simulink model "FrankSensingDiscreteEKF"  (R2025a)
settings: Solver=FixedStepAuto  StartTime=0.0  StopTime=150  FixedStep=.001  RelTol=1e-3
model workspace (MAT data in the model file):
  GPSvehyUpdate = 0
libraries: simulink x1
(part 1 of 2)
settings Model: SimulationMode=rapid-accelerator  Creator=ncpet  LastModifiedBy=ncpet
settings RTWCC: GPUComputeCapability=3.5

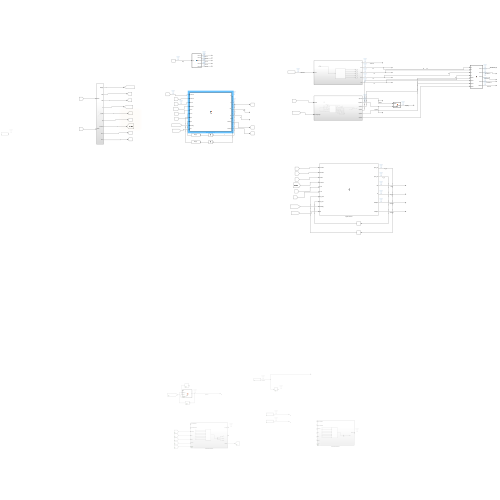
[thumbnail: Simulink's stored preview of the top-level diagram]
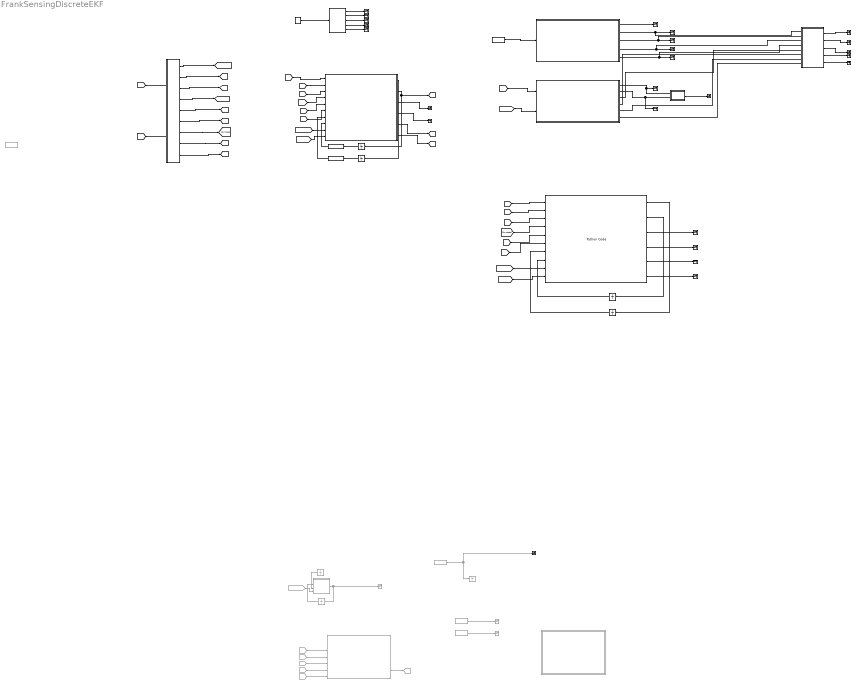
== system FrankSensingDiscreteEKF ==
  From Workspace : FromWorkspace  VariableName=LatAccel
  From Workspace4 : FromWorkspace  Commented=on  VariableName=X
  From Workspace5 : FromWorkspace  Commented=on  VariableName=Y
  From Workspace6 : FromWorkspace  Commented=on  VariableName=SteeringAngle
  From Workspace8 : FromWorkspace  Commented=on  VariableName=TicksYR
  From14 : From  Commented=on  GotoTag=startflag
  From3 : From  Commented=on  GotoTag=Vvehx
  From4 : From  Commented=on  GotoTag=Steerangle
  From5 : From  Commented=on  GotoTag=Psid
  From6 : From  Commented=on  GotoTag=Xcov
  From7 : From  Commented=on  GotoTag=Ycov
  Goto5 : Goto  Commented=on  GotoTag=Rbias
  Integrator1 : Integrator  Commented=on
  MATLAB Function : MATLAB Function  Commented=on  TreatAsAtomicUnit=on
  MATLAB Function1 : MATLAB Function  TreatAsAtomicUnit=on
  MATLAB Function2 : MATLAB Function  TreatAsAtomicUnit=on
  MATLAB Function3 : MATLAB Function  TreatAsAtomicUnit=on
  MATLAB Function4 : MATLAB Function  TreatAsAtomicUnit=on
  Python Code1 : PythonCode  InitializeConditionsCode=|  OutputCode=|  TerminateCode=pass  SampleTime=.001
      InitializeConditionsCode=|
      | import numpy as np
      | 
      | # Initial state vector  [Vy, Vx, r, Psi, Ax, Rbias, Abias]
      | Xpri_init = np.array([0.5, -1.9, -0.49, 0.0, 0.34, -0.022, -0.2], dtype=float)
      | 
      | # Initial covariance (7x7 diagonal), flattened row-major
      | P_init_diag = np.diag([0.1, 0.1, 0.1, 0.1, 0.001, 0.001, 0.001])
      | Ppri_init   = P_init_diag.flatten()   # 49 values
      OutputCode=|
      | import numpy as np
      | import EKFfcn2
      | 
      | u = [VYmeas, VXmeas, rmeas, Axmeas,
      |      Xcov, Ycov,
      |      *Ppri_flat,   # 49 values (7x7 flattened)
      |      *Xpri_arr,    # 7 values
      |      startflag,
      |      SA]
      | 
      | y = EKFfcn2.simulink_step(u)
      | 
      | # Unpack outputs
      | Ppri_out  = y[0:49]    # 7x7 covariance, flattened
      | Xpri_out  = y[49:56]   # 7 states
      | res       = y[56:60]   # 4 residuals
      | fk        = y[60:67]   # 7 predicted states
      | Rbiaspri  = y[67]
      | Abiaspri  = y[68]
  Ramp : simulink/Sources/Ramp  slope=.1  start=0  InitialOutput=.001
  Signal Specification : SignalSpecification  Dimensions=[7 7]
  Signal Specification1 : SignalSpecification  Dimensions=[7 1]
  State Estimation : Subsystem  Commented=on
  State Estimation1 : Subsystem  Commented=on
  Subsystem1 : Subsystem
  Subsystem3 : Subsystem
  Subsystem4 : Subsystem
  Terminator : Terminator  Commented=on
  Terminator{1..2,5..23,29..32} (25 alike) : Terminator
  Terminator3 : Terminator  Commented=on
  Terminator4 : Terminator  Commented=on
  Unit Delay : UnitDelay  Commented=on  SampleTime=-1  HasFrameUpgradeWarning=on
  Unit Delay1 : UnitDelay  Commented=on  SampleTime=-1  HasFrameUpgradeWarning=on
  Unit Delay2 : UnitDelay  SampleTime=-1  HasFrameUpgradeWarning=on
  Unit Delay3 : UnitDelay  InitialCondition=[.1 0 0 0 0 0 0, 0 .1 0 0 0 0 0, 0 0 .1 0 0 0 0, 0 0 0 .1 0 0 0, 0 0 0 0 .001 0 0, 0 0 0 0 0 .001 0, 0 0 0 0 0 0 .001]  SampleTime=.001  HasFrameUpgradeWarning=on
  Unit Delay4 : UnitDelay  SampleTime=-1  HasFrameUpgradeWarning=on
  Unit Delay5 : UnitDelay  InitialCondition=[.5, -1.9, -.49, 0, .34, -.022, -.2]  SampleTime=.001  HasFrameUpgradeWarning=on
  wires:
  From Workspace4/1 -> Terminator3/1  "x"
  From Workspace5/1 -> Terminator4/1  "y"
  From Workspace8/1 -> Integrator1/1, Terminator13/1  "TicksYR"
  From3/1 -> State Estimation/4(Vx)
  From4/1 -> State Estimation/5(SA)
  From5/1 -> State Estimation/3(rmeas)
  From6/1 -> State Estimation/6(Xcov)
  From7/1 -> State Estimation/7(Ycov)
  State Estimation/3(Rbias) -> Goto5/1
  MATLAB Function/1(x) -> Terminator/1, Unit Delay/1  "psiNum"
  Unit Delay/1 -> MATLAB Function/2(Xdpri)
  From14/1 -> MATLAB Function/4(startflag)
  Unit Delay1/1 -> MATLAB Function/3(Xpri)
  Subsystem1/1(Slipflag) -> [startflag]
  Subsystem1/2(XdS) -> [Xd]
  Subsystem1/3(YdS) -> [Yd]
  Subsystem1/4(Out4) -> [Steerangle]
  Subsystem1/5(PsidS) -> [Psid]
  Subsystem1/6(psi) -> [psi]
  Subsystem1/7(Axmeas) -> [Axmeas]
  Subsystem1/8(Xcov) -> [Xcov]
  Subsystem1/9(Ycov) -> [Ycov]
  [Xcov] -> MATLAB Function1/5(Xcov)
  [Ycov] -> MATLAB Function1/6(Ycov)
  MATLAB Function1/2(X) -> Unit Delay2/1, [States]  "X"
  Unit Delay2/1 -> Signal Specification1/1
  MATLAB Function1/1(P) -> Unit Delay4/1  "Pmat"
  Unit Delay4/1 -> Signal Specification/1
  [Axmeas] -> MATLAB Function1/4(Axmeas)
  [Xd] -> MATLAB Function1/2(VXmeas)
  [startflag] -> MATLAB Function1/9(startflag)
  [Steerangle] -> MATLAB Function1/10(SA)
  Signal Specification/1 -> MATLAB Function1/7(Ppri)
  Signal Specification1/1 -> MATLAB Function1/8(Xpri)
  MATLAB Function1/3(res) -> Terminator1/1  "res"
  MATLAB Function1/4(fk) -> Terminator2/1  "fk"
  [States] -> Subsystem3/1(States)
  [Steerangle] -> Subsystem3/2(SteeringAngle)
  Subsystem3/1(AlphaF) -> MATLAB Function2/1(AlphaF), Terminator5/1  "AlphaF"
  Subsystem3/2(AlphaR) -> Terminator8/1, MATLAB Function2/2(AlphaR)  "AlphaR"
  MATLAB Function2/1(SlipMag) -> Terminator10/1  "SlipMag"
  From Workspace/1 -> Subsystem4/1(Accel)  "LatAccel"
  Subsystem4/1(Outport) -> Terminator11/1  "TireForce"
  MATLAB Function1/5(Rbiaspri) -> [Rbias]
  [Rbias] -> Subsystem1/1(Rbias)
  MATLAB Function1/6(Abiaspri) -> [Abiaspri]
  [Abiaspri] -> Subsystem1/2(Abias)
  Ramp/1 -> MATLAB Function3/1(slip)  "Slip"
  MATLAB Function3/1(Force1) -> Terminator14/1  "Force1"
  MATLAB Function3/2(Force2) -> Terminator15/1  "Force2"
  MATLAB Function3/3(Force3) -> Terminator16/1  "Force3"
  MATLAB Function3/5(Force5) -> Terminator18/1  "Force5"
  MATLAB Function3/4(Force4) -> Terminator17/1  "Force4"
  Subsystem3/5(Alpha4) -> MATLAB Function4/7(Alpha4)
  Subsystem4/3(Ffl) -> MATLAB Function4/2(Ffl), Terminator7/1  "Ffl"
  MATLAB Function4/5(TotForce) -> Terminator23/1  "TotForce"
  MATLAB Function4/2(Force2) -> Terminator20/1  "FflLatForce"
  Subsystem3/4(Alpha3) -> MATLAB Function4/6(Alpha3)
  Subsystem4/4(Frr) -> MATLAB Function4/3(Frr), Terminator9/1  "Frr"
  Subsystem3/6(Alpha5) -> MATLAB Function4/8(Alpha5)
  Subsystem3/3(Alpha2) -> MATLAB Function4/5(Alpha2)
  MATLAB Function4/4(Force4) -> Terminator22/1  "FrlLatForce"
  MATLAB Function4/1(Force1) -> Terminator19/1  "FfrLatForce"
  Subsystem4/5(Frl) -> MATLAB Function4/4(Frl), Terminator12/1  "Frl"
  Subsystem4/2(Ffr) -> MATLAB Function4/1(Ffr), Terminator6/1  "Ffr"
  MATLAB Function4/3(Force3) -> Terminator21/1  "FrrLatForce"
  Unit Delay3/1 -> Python Code1/7
  Python Code1/1 -> Unit Delay3/1  "P_py"
  Python Code1/2 -> Unit Delay5/1  "X_py"
  Unit Delay5/1 -> Python Code1/8
  [startflag] -> Python Code1/9
  Python Code1/6 -> Terminator32/1  "AbiasPY"
  Python Code1/5 -> Terminator31/1  "RbiasPY"
  Python Code1/4 -> Terminator30/1  "fk_py"
  Python Code1/3 -> Terminator29/1  "resPY"
  [Axmeas] -> Python Code1/4
  [Psid] -> Python Code1/3
  [Xd] -> Python Code1/2
  [Ycov] -> Python Code1/6
  [Xcov] -> Python Code1/5
  [Yd] -> Python Code1/1
  [Steerangle] -> Python Code1/10
  [Yd] -> MATLAB Function1/1(VYmeas)
  [Psid] -> MATLAB Function1/3(rmeas)

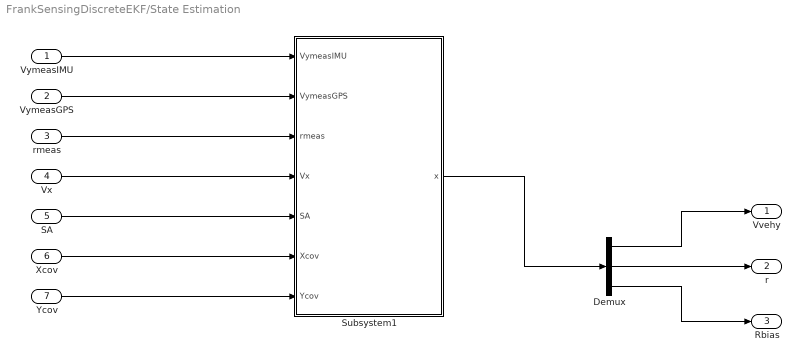
== system FrankSensingDiscreteEKF/State Estimation ==
  VymeasIMU : Inport
  VymeasGPS : Inport  Port=2
  rmeas : Inport  Port=3
  Vx : Inport  Port=4
  SA : Inport  Port=5
  Xcov : Inport  Port=6
  Ycov : Inport  Port=7
  Demux : Demux  Outputs=3
  Subsystem1 : Subsystem
  Vvehy : Outport
  r : Outport  Port=2
  Rbias : Outport  Port=3
  wires:
  VymeasIMU/1 -> Subsystem1/1(VymeasIMU)
  VymeasGPS/1 -> Subsystem1/2(VymeasGPS)
  rmeas/1 -> Subsystem1/3(rmeas)
  Vx/1 -> Subsystem1/4(Vx)
  SA/1 -> Subsystem1/5(SA)
  Subsystem1/1(x) -> Demux/1
  Demux/1 -> Vvehy/1
  Xcov/1 -> Subsystem1/6(Xcov)
  Ycov/1 -> Subsystem1/7(Ycov)
  Demux/2 -> r/1
  Demux/3 -> Rbias/1

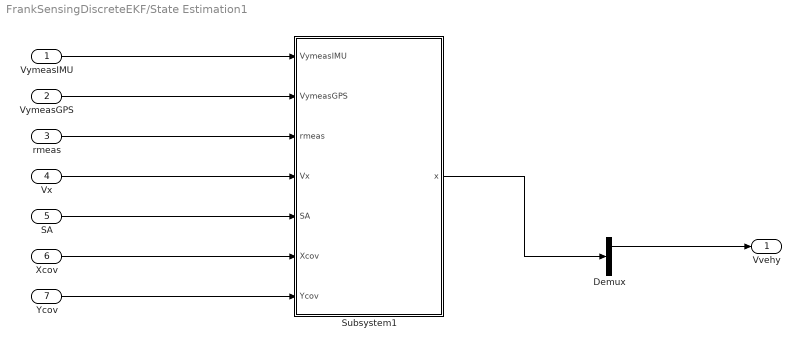
== system FrankSensingDiscreteEKF/State Estimation1 ==
  VymeasIMU : Inport
  VymeasGPS : Inport  Port=2
  rmeas : Inport  Port=3
  Vx : Inport  Port=4
  SA : Inport  Port=5
  Xcov : Inport  Port=6
  Ycov : Inport  Port=7
  Demux : Demux  Outputs=2
  Subsystem1 : Subsystem
  Vvehy : Outport
  wires:
  Ycov/1 -> Subsystem1/7(Ycov)
  Xcov/1 -> Subsystem1/6(Xcov)
  Demux/1 -> Vvehy/1
  Subsystem1/1(x) -> Demux/1
  SA/1 -> Subsystem1/5(SA)
  Vx/1 -> Subsystem1/4(Vx)
  rmeas/1 -> Subsystem1/3(rmeas)
  VymeasGPS/1 -> Subsystem1/2(VymeasGPS)
  VymeasIMU/1 -> Subsystem1/1(VymeasIMU)

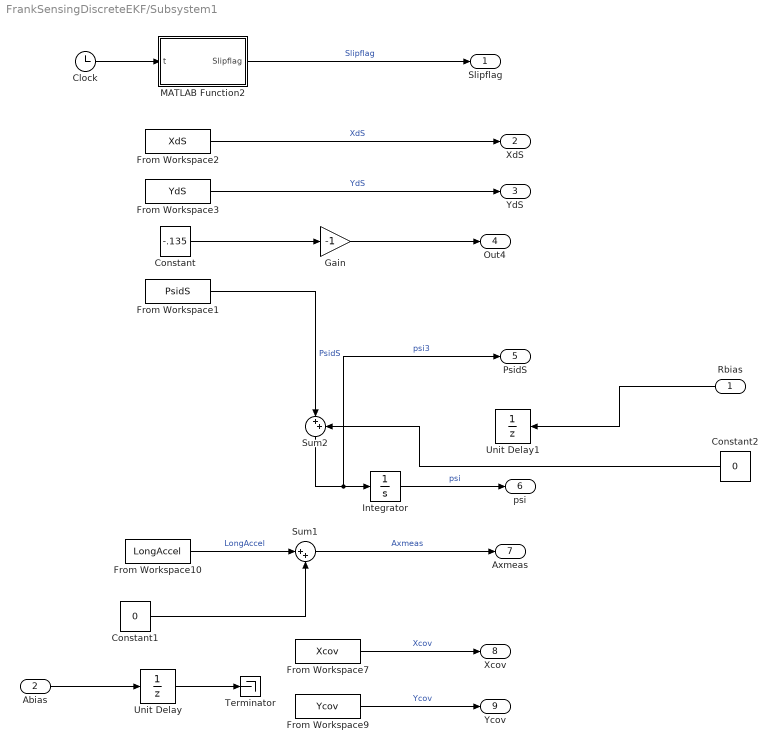
== system FrankSensingDiscreteEKF/Subsystem1 ==
  Rbias : Inport
  Abias : Inport  Port=2
  Clock : Clock
  Constant : Constant  Value=-.135
  Constant1 : Constant  Value=0
  Constant2 : Constant  Value=0
  From Workspace1 : FromWorkspace  VariableName=PsidS
  From Workspace10 : FromWorkspace  VariableName=LongAccel
  From Workspace2 : FromWorkspace  VariableName=XdS
  From Workspace3 : FromWorkspace  VariableName=YdS
  From Workspace7 : FromWorkspace  VariableName=Xcov
  From Workspace9 : FromWorkspace  VariableName=Ycov
  Gain : Gain  Gain=-1
  Integrator : Integrator
  MATLAB Function2 : MATLAB Function  TreatAsAtomicUnit=on
  Sum1 : Sum  Inputs=|++
  Sum2 : Sum  Inputs=|++
  Terminator : Terminator
  Unit Delay : UnitDelay  SampleTime=-1  HasFrameUpgradeWarning=on
  Unit Delay1 : UnitDelay  SampleTime=-1  HasFrameUpgradeWarning=on
  Slipflag : Outport
  XdS : Outport  Port=2
  YdS : Outport  Port=3
  Out4 : Outport  Port=4
  PsidS : Outport  Port=5
  psi : Outport  Port=6
  Axmeas : Outport  Port=7
  Xcov : Outport  Port=8
  Ycov : Outport  Port=9
  wires:
  From Workspace1/1 -> Sum2/1  "PsidS"
  From Workspace7/1 -> Xcov/1  "Xcov"
  Constant/1 -> Gain/1
  Sum2/1 -> PsidS/1, Integrator/1  "psi3"
  From Workspace10/1 -> Sum1/1  "LongAccel"
  Clock/1 -> MATLAB Function2/1(t)
  From Workspace9/1 -> Ycov/1  "Ycov"
  From Workspace2/1 -> XdS/1  "XdS"
  From Workspace3/1 -> YdS/1  "YdS"
  Integrator/1 -> psi/1  "psi"
  Sum1/1 -> Axmeas/1  "Axmeas"
  MATLAB Function2/1(Slipflag) -> Slipflag/1  "Slipflag"
  Abias/1 -> Unit Delay/1
  Rbias/1 -> Unit Delay1/1
  Gain/1 -> Out4/1
  Constant1/1 -> Sum1/2
  Unit Delay/1 -> Terminator/1
  Constant2/1 -> Sum2/2

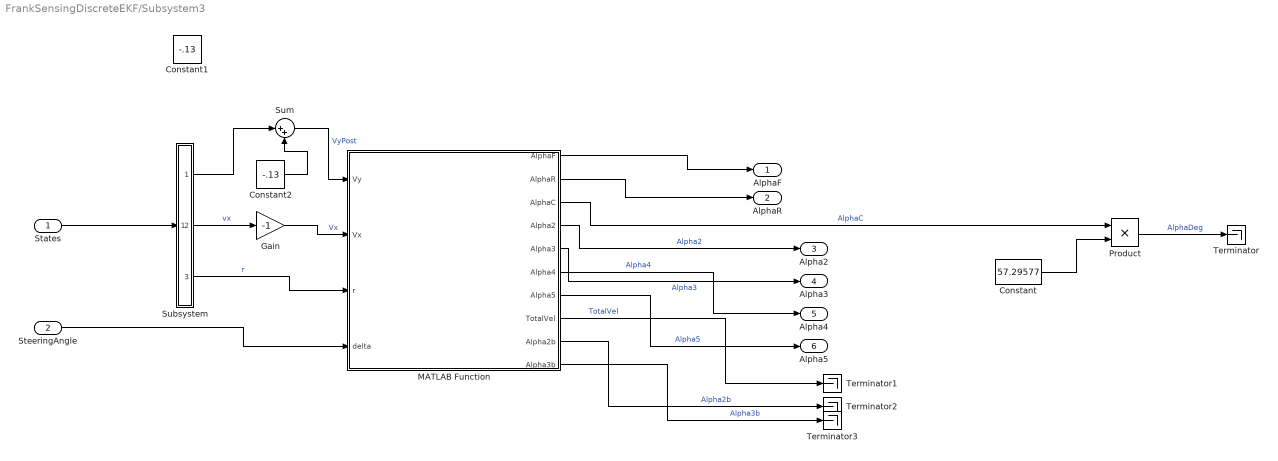
== system FrankSensingDiscreteEKF/Subsystem3 ==
  States : Inport
  SteeringAngle : Inport  Port=2
  Constant : Constant  Value=57.29577
  Constant1 : Constant  Value=-.13
  Constant2 : Constant  Value=-.13
  Gain : Gain  Gain=-1
  MATLAB Function : MATLAB Function  TreatAsAtomicUnit=on
  Product : Product
  Subsystem : Subsystem
  Sum : Sum  Inputs=|++
  Terminator{,1..3} (4 alike) : Terminator
  AlphaF : Outport
  AlphaR : Outport  Port=2
  Alpha2 : Outport  Port=3
  Alpha3 : Outport  Port=4
  Alpha4 : Outport  Port=5
  Alpha5 : Outport  Port=6
  wires:
  States/1 -> Subsystem/1(In1)
  Subsystem/2(Out2) -> Gain/1  "vx"
  Subsystem/3(Out3) -> MATLAB Function/3(r)  "r"
  SteeringAngle/1 -> MATLAB Function/4(delta)
  MATLAB Function/2(AlphaR) -> AlphaR/1
  MATLAB Function/1(AlphaF) -> AlphaF/1
  MATLAB Function/3(AlphaC) -> Product/1  "AlphaC"
  Constant/1 -> Product/2
  Product/1 -> Terminator/1  "AlphaDeg"
  MATLAB Function/4(Alpha2) -> Alpha2/1  "Alpha2"
  MATLAB Function/5(Alpha3) -> Alpha3/1  "Alpha3"
  MATLAB Function/6(Alpha4) -> Alpha4/1  "Alpha4"
  MATLAB Function/7(Alpha5) -> Alpha5/1  "Alpha5"
  MATLAB Function/8(TotalVel) -> Terminator1/1  "TotalVel"
  MATLAB Function/9(Alpha2b) -> Terminator2/1  "Alpha2b"
  MATLAB Function/10(Alpha3b) -> Terminator3/1  "Alpha3b"
  Gain/1 -> MATLAB Function/2(Vx)  "Vx"
  Subsystem/1(Out1) -> Sum/1
  Sum/1 -> MATLAB Function/1(Vy)  "VyPost"
  Constant2/1 -> Sum/2

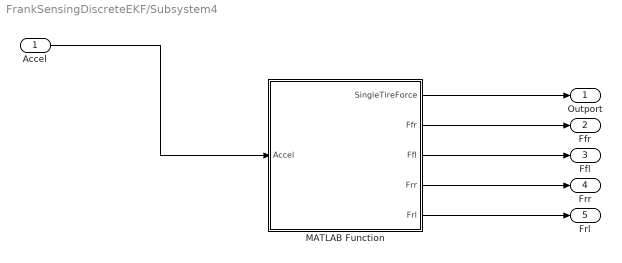
== system FrankSensingDiscreteEKF/Subsystem4 ==
  Accel : Inport
  MATLAB Function : MATLAB Function  TreatAsAtomicUnit=on
  Outport : Outport
  Ffr : Outport  Port=2
  Ffl : Outport  Port=3
  Frr : Outport  Port=4
  Frl : Outport  Port=5
  wires:
  Accel/1 -> MATLAB Function/1(Accel)
  MATLAB Function/1(SingleTireForce) -> Outport/1
  MATLAB Function/2(Ffr) -> Ffr/1
  MATLAB Function/3(Ffl) -> Ffl/1
  MATLAB Function/4(Frr) -> Frr/1
  MATLAB Function/5(Frl) -> Frl/1

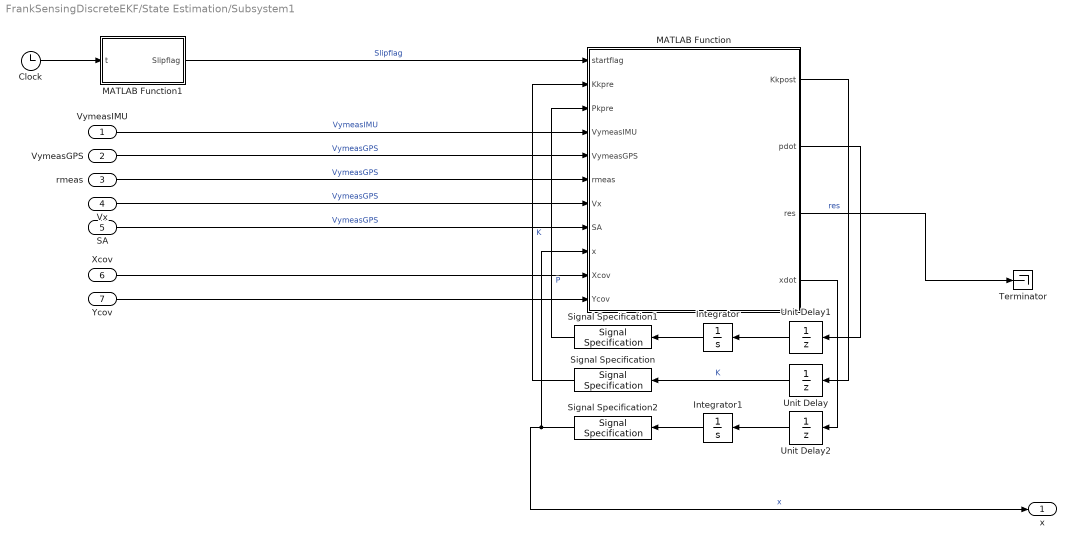
== system FrankSensingDiscreteEKF/State Estimation/Subsystem1 ==
  VymeasIMU : Inport
  VymeasGPS : Inport  Port=2
  rmeas : Inport  Port=3
  Vx : Inport  Port=4
  SA : Inport  Port=5
  Xcov : Inport  Port=6
  Ycov : Inport  Port=7
  Clock : Clock
  Integrator : Integrator  InitialCondition=[.001 0 0;0 .001 0;0 0 .001]
  Integrator1 : Integrator  InitialCondition=[-0.014;-0.44;-.022]
  MATLAB Function : MATLAB Function  TreatAsAtomicUnit=on
  MATLAB Function1 : MATLAB Function  TreatAsAtomicUnit=on
  Signal Specification : SignalSpecification  Dimensions=[3 3]
  Signal Specification1 : SignalSpecification  Dimensions=[3 3]
  Signal Specification2 : SignalSpecification  Dimensions=[3 1]
  Terminator : Terminator
  Unit Delay : UnitDelay  SampleTime=-1  HasFrameUpgradeWarning=on
  Unit Delay1 : UnitDelay  SampleTime=-1  HasFrameUpgradeWarning=on
  Unit Delay2 : UnitDelay  SampleTime=-1  HasFrameUpgradeWarning=on
  x : Outport
  wires:
  MATLAB Function/1(Kkpost) -> Unit Delay/1
  Signal Specification/1 -> MATLAB Function/2(Kkpre)  "K"
  MATLAB Function/2(pdot) -> Unit Delay1/1
  Integrator/1 -> Signal Specification1/1
  Unit Delay/1 -> Signal Specification/1  "K"
  Unit Delay1/1 -> Integrator/1
  Signal Specification1/1 -> MATLAB Function/3(Pkpre)  "P"
  VymeasIMU/1 -> MATLAB Function/4(VymeasIMU)  "VymeasIMU"
  MATLAB Function/3(res) -> Terminator/1  "res"
  VymeasGPS/1 -> MATLAB Function/5(VymeasGPS)  "VymeasGPS"
  rmeas/1 -> MATLAB Function/6(rmeas)  "VymeasGPS"
  Vx/1 -> MATLAB Function/7(Vx)  "VymeasGPS"
  Clock/1 -> MATLAB Function1/1(t)
  MATLAB Function1/1(Slipflag) -> MATLAB Function/1(startflag)  "Slipflag"
  SA/1 -> MATLAB Function/8(SA)  "VymeasGPS"
  MATLAB Function/4(xdot) -> Unit Delay2/1
  Unit Delay2/1 -> Integrator1/1
  Integrator1/1 -> Signal Specification2/1
  Signal Specification2/1 -> x/1, MATLAB Function/9(x)  "x"
  Xcov/1 -> MATLAB Function/10(Xcov)
  Ycov/1 -> MATLAB Function/11(Ycov)

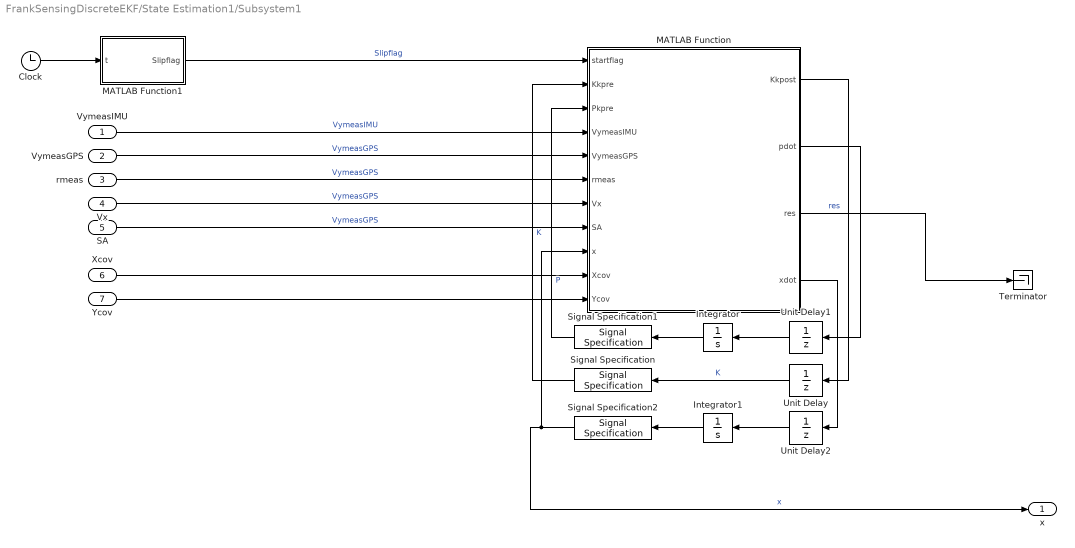
== system FrankSensingDiscreteEKF/State Estimation1/Subsystem1 ==
  VymeasIMU : Inport
  VymeasGPS : Inport  Port=2
  rmeas : Inport  Port=3
  Vx : Inport  Port=4
  SA : Inport  Port=5
  Xcov : Inport  Port=6
  Ycov : Inport  Port=7
  Clock : Clock
  Integrator : Integrator  InitialCondition=[.001 0;0 .001]
  Integrator1 : Integrator  InitialCondition=[-0.014;-0.44]
  MATLAB Function : MATLAB Function  TreatAsAtomicUnit=on
  MATLAB Function1 : MATLAB Function  TreatAsAtomicUnit=on
  Signal Specification : SignalSpecification  Dimensions=[2 3]
  Signal Specification1 : SignalSpecification  Dimensions=[2 2]
  Signal Specification2 : SignalSpecification  Dimensions=[2 1]
  Terminator : Terminator
  Unit Delay : UnitDelay  SampleTime=-1  HasFrameUpgradeWarning=on
  Unit Delay1 : UnitDelay  SampleTime=-1  HasFrameUpgradeWarning=on
  Unit Delay2 : UnitDelay  SampleTime=-1  HasFrameUpgradeWarning=on
  x : Outport
  wires:
  Ycov/1 -> MATLAB Function/11(Ycov)
  Xcov/1 -> MATLAB Function/10(Xcov)
  Signal Specification2/1 -> MATLAB Function/9(x), x/1  "x"
  Integrator1/1 -> Signal Specification2/1
  Unit Delay2/1 -> Integrator1/1
  MATLAB Function/4(xdot) -> Unit Delay2/1
  SA/1 -> MATLAB Function/8(SA)  "VymeasGPS"
  MATLAB Function1/1(Slipflag) -> MATLAB Function/1(startflag)  "Slipflag"
  Clock/1 -> MATLAB Function1/1(t)
  Vx/1 -> MATLAB Function/7(Vx)  "VymeasGPS"
  rmeas/1 -> MATLAB Function/6(rmeas)  "VymeasGPS"
  VymeasGPS/1 -> MATLAB Function/5(VymeasGPS)  "VymeasGPS"
  MATLAB Function/3(res) -> Terminator/1  "res"
  VymeasIMU/1 -> MATLAB Function/4(VymeasIMU)  "VymeasIMU"
  Signal Specification1/1 -> MATLAB Function/3(Pkpre)  "P"
  Unit Delay1/1 -> Integrator/1
  Unit Delay/1 -> Signal Specification/1  "K"
  Integrator/1 -> Signal Specification1/1
  MATLAB Function/2(pdot) -> Unit Delay1/1
  Signal Specification/1 -> MATLAB Function/2(Kkpre)  "K"
  MATLAB Function/1(Kkpost) -> Unit Delay/1

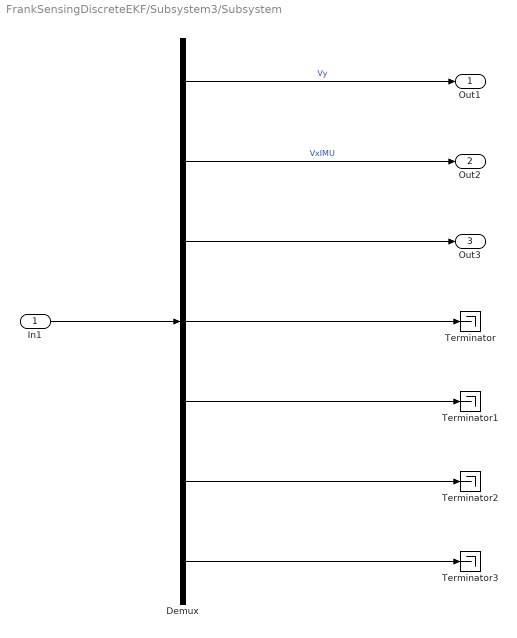
== system FrankSensingDiscreteEKF/Subsystem3/Subsystem ==
  In1 : Inport
  Demux : Demux  Outputs=7
  Terminator{,1..3} (4 alike) : Terminator
  Out1 : Outport
  Out2 : Outport  Port=2
  Out3 : Outport  Port=3
  wires:
  In1/1 -> Demux/1
  Demux/3 -> Out3/1
  Demux/2 -> Out2/1  "VxIMU"
  Demux/1 -> Out1/1  "Vy"
  Demux/4 -> Terminator/1
  Demux/5 -> Terminator1/1
  Demux/6 -> Terminator2/1
  Demux/7 -> Terminator3/1

== matlab function FrankSensingDiscreteEKF/State Estimation1/Subsystem1/MATLAB Function1 ==
  data: t input; Slipflag output
function Slipflag = fcn(t)

if t == 0
    Slipflag = 0;
else
    Slipflag = 1;
end

t

== matlab function FrankSensingDiscreteEKF/Subsystem3/MATLAB Function ==
  data: Vy input; AlphaF output; Vx input; r input; delta input; AlphaR output; AlphaC output; Alpha2 output; Alpha3 output; Alpha4 output; Alpha5 output; TotalVel output; Alpha2b output; Alpha3b output
function [AlphaF,AlphaR,AlphaC,Alpha2,Alpha3,Alpha4,Alpha5,TotalVel,Alpha2b,Alpha3b] = fcn(Vy,Vx, r,delta)

a = .3036;
b = .2484;
P21xhat = .3036;
P31xhat = .3036;
P41xhat = .2484;
P51xhat = .2484;

P21yhat = .20955;
P31yhat = .20955;
P41yhat = .20955;
P51yhat = .20955;

% B = 10;
% C = 1.6;
% D = 73.1580;
% E = 1;
% Iz = 1;
% Mv = 15.7;
% delta = SA;
% Ts = 0.01;

% AlphaF = atan((-Vy+a*(r))/Vx)+delta;
% AlphaR = atan((-Vy-b*(r))/Vx);
AlphaF =  delta - (-Vy+a*r)/Vx;
AlphaR = -(-Vy-b*r)/Vx;
AlphaC = -atan(-Vy/Vx);
TotalVel = sqrt((Vx^2+Vy^2));

LatRefvelfr = (-Vy+P21xhat*r)/(Vx+P21yhat*r);
LatRefvelfl = (-Vy+P31xhat*r)/(Vx-P31yhat*r);
LatRefvelrr = (-Vy-P41xhat*r)/(Vx+P41yhat*r);
LatRefvelrl = (-Vy-P51xhat*r)/(Vx-P51yhat*r);
% 
Alpha2 = delta - atan(LatRefvelfr);%+delta;
Alpha3 = delta - atan(LatRefvelfl);%+delta;
Alpha2b = atan(LatRefvelfr);
Alpha3b = atan(LatRefvelfl);
Alpha4 = -(atan(LatRefvelrr));
Alpha5 = -(atan(LatRefvelrl));
Alphas = [Alpha2;Alpha3;Alpha4;Alpha5];

== matlab function FrankSensingDiscreteEKF/Subsystem1/MATLAB Function2 ==
  data: t input; Slipflag output
function Slipflag = fcn(t)

if t == 0
    Slipflag = 0;
else
    Slipflag = 1;
end

t

== matlab function FrankSensingDiscreteEKF/MATLAB Function ==
  data: Xd input; x output; Xdpri input; Xpri input; startflag input
function x = fcn(Xd,Xdpri,Xpri,startflag)

if startflag == 0
    Xdpri = 0;
    Xpri = 0;
else
    Xdpri = Xdpri;
    Xpri = Xpri;
end

x = Xpri + (.001/2)*(Xd+Xdpri);

== matlab function FrankSensingDiscreteEKF/MATLAB Function2 ==
  data: AlphaF input; SlipMag output; AlphaR input
function SlipMag = fcn(AlphaF, AlphaR)

SlipMag = sqrt((AlphaF)^2+(AlphaR)^2);

== matlab function FrankSensingDiscreteEKF/State Estimation/Subsystem1/MATLAB Function ==
  data: startflag input; Kkpre input; Pkpre input; VymeasIMU input; Kkpost output; pdot output; VymeasGPS input; rmeas input; res output; Vx input; SA input; x input; xdot output; Xcov input; Ycov input
function [Kkpost, pdot, res, xdot] = myEKF(startflag, Kkpre, Pkpre, VymeasIMU, VymeasGPS, rmeas, Vx, SA, x, Xcov, Ycov)

a = .3036;
b = .2484;
B = 10;
C = 1.6;
D = 73.1580;
E = 1;
Iz = 1;
Mv = 15.7;
delta = SA;




VyvarIMU = 200;
VyvarGPS = Xcov;
rvar = .00001;


Rk = [VyvarIMU 0          0;...     
      0        VyvarGPS   0;...
      0        0          rvar];  %Measurement noise covariance matrix
      

Qk = [.1     0      0;...
      0     .1      0;...
      0      0      .1]; % process noise covariance matrix

zk = [VymeasIMU; VymeasGPS; rmeas];


% Startup Initialization
if startflag == 0
    Kk = [0    0  0;...
          0    0  0;...
          0    0  0];
    Pk = [.00001     0          0;...
          0          .000002    0;...
          0          0          .000003]; 

    x = [-0.014;-0.44;-.022];
      
else
    Kk = Kkpre
    Pk = Pkpre
end

hk = [x(1);x(1);x(2)];
Vy = x(1);
r = x(2);
Rbias = x(3);
% Prediction and measurement jacobian
Hk = [1 0 0;1 0 0;0 1 0];

Fkf = Fk(B,C,D,E,Iz,Mv,Rbias,Vx,Vy,a,b,delta,r);
fkf = Xdot(B,C,D,E,Iz,Mv,Rbias,Vx,Vy,a,b,delta,r);
res = zk-hk;
xdot = fkf+Kk*(res);
pdot = Fkf*Pk+Pk*Fkf'-Kk*Hk*Pk+Qk;
Kkpost = Pk*Hk'*inv(Rk);





% % Measurement Updates
% S = (Hk*Pk*Hk')+Rk;
% Kkpost = Pk*Hk'*inv(S)
% Pkpost = Pk-Kk*Hk*Pk
% res = zk-Hk
% xhat = Statest + Kkpost*(res)
% 
% % % State Estimate update
% pdot = Fkf'*Pkpost+Pkpost*Fkf'-Kkpost*Hk*Pkpost + Qk

== matlab function FrankSensingDiscreteEKF/Subsystem4/MATLAB Function ==
  data: Accel input; SingleTireForce output; Ffr output; Ffl output; Frr output; Frl output
function [SingleTireForce, Ffr, Ffl, Frr, Frl] = fcn(Accel)

Mv = 15.76;
c = .20955;

a = .3036;
b = .2484;
L = .093375;
g = 9.81;

SingleTireForce = Mv*Accel;

Frr = (Mv*g*a)/(2*(a+b))-(.5*Mv*Accel*L*a)/(c*(a+b));
Frl = (Mv*g*a)/(2*(a+b))+(.5*Mv*Accel*L*a)/(c*(a+b));
Ffr = (Mv*g*b)/(2*(a+b))-(.5*Mv*Accel*L*b)/(c*(a+b));
Ffl = (Mv*g*b)/(2*(a+b))+(.5*Mv*Accel*L*b)/(c*(a+b));

== matlab function FrankSensingDiscreteEKF/MATLAB Function4 ==
  data: Ffr input; Ffl input; Frr input; Frl input; Force1 output; Alpha2 input; Alpha3 input; Alpha4 input; Alpha5 input; Force2 output; Force3 output; Force4 output; TotForce output
function [Force1,Force2,Force3,Force4,TotForce] = fcn(Ffr,Ffl,Frr,Frl,Alpha2,Alpha3,Alpha4,Alpha5)
a1 = .8;
a2 = .001;
a3 = 1.05;
a4 = 185;
a5 = .6;
a6 = 6;
a7 = -.003;
a8 = 0;
a9 = .707;
Ffr1 = Ffr
Ffl1 = Ffl
Frr1 = Frr
Frl1 = Frl
slip1 = Alpha2
slip2 = Alpha3
slip3 = Alpha4
slip4 = Alpha5
Force1 = ((a2*Ffr1.^2+a3*Ffr1).*sin(a1*atan(((a4*sin(a5*atan(a6*Ffr1)))./((a2*Ffr1.^2+a3*Ffr1)*a1)).*((a1-(a7*Ffr1.^2+a8*Ffr1+a9)).*slip1 + ((a7*Ffr1.^2+a8*Ffr1+a9)./((a4*sin(a5*atan(a6*Ffr1)))./((a2*Ffr1.^2+a3*Ffr1)*a1))).*atan(((a4*sin(a5*atan(a6*Ffr1)))./((a2*Ffr1.^2+a3*Ffr1)*a1)).*slip1)))));
Force2 = ((a2*Ffl1.^2+a3*Ffl1).*sin(a1*atan(((a4*sin(a5*atan(a6*Ffl1)))./((a2*Ffl1.^2+a3*Ffl1)*a1)).*((a1-(a7*Ffl1.^2+a8*Ffl1+a9)).*slip2 + ((a7*Ffl1.^2+a8*Ffl1+a9)./((a4*sin(a5*atan(a6*Ffl1)))./((a2*Ffl1.^2+a3*Ffl1)*a1))).*atan(((a4*sin(a5*atan(a6*Ffl1)))./((a2*Ffl1.^2+a3*Ffl1)*a1)).*slip2)))));
Force3 = ((a2*Frr1.^2+a3*Frr1).*sin(a1*atan(((a4*sin(a5*atan(a6*Frr1)))./((a2*Frr1.^2+a3*Frr1)*a1)).*((a1-(a7*Frr1.^2+a8*Frr1+a9)).*slip3 + ((a7*Frr1.^2+a8*Frr1+a9)./((a4*sin(a5*atan(a6*Frr1)))./((a2*Frr1.^2+a3*Frr1)*a1))).*atan(((a4*sin(a5*atan(a6*Frr1)))./((a2*Frr1.^2+a3*Frr1)*a1)).*slip3)))));
Force4 = ((a2*Frl1.^2+a3*Frl1).*sin(a1*atan(((a4*sin(a5*atan(a6*Frl1)))./((a2*Frl1.^2+a3*Frl1)*a1)).*((a1-(a7*Frl1.^2+a8*Frl1+a9)).*slip4 + ((a7*Frl1.^2+a8*Frl1+a9)./((a4*sin(a5*atan(a6*Frl1)))./((a2*Frl1.^2+a3*Frl1)*a1))).*atan(((a4*sin(a5*atan(a6*Frl1)))./((a2*Frl1.^2+a3*Frl1)*a1)).*slip4)))));
TotForce = Force1+Force2+Force3+Force4

== matlab function FrankSensingDiscreteEKF/MATLAB Function3 ==
  data: slip input; Force1 output; Force2 output; Force3 output; Force4 output; Force5 output
function [Force1,Force2,Force3,Force4,Force5] = fcn( slip)
Ffr1 = 50
Ffr2 = 45
Ffr3 = 40
Ffr4 = 35
Ffr5 = 30
a1 = .8;
a2 = .001;
a3 = 1.05;
a4 = 185;
a5 = .6;
a6 = 6;
a7 = -.003;
a8 = 0;
a9 = .707;
% a1 = .9;
% a2 = .001;
% a3 = 1.35;
% a4 = 125;
% a5 = .6;
% a6 = 6;
% a7 = -.002;
% a8 = 0;
% a9 = .707;
% a1 = .9918;
% a2 = .001;
% a3 = 1.116;
% a4 = 109.53;
% a5 = 1.74;
% a6 = 385.37;
% a7 = -23.87;
% a8 = 9;
% a9 = 2.6;
% a1 = .2317;
% a2 = -.0631;
% a3 = -.0043;
% a4 = 1398;
% a5 = 1.9811;
% a6 = 2183;
% a7 = -131.4390;
% a8 = 3435;
% a9 = 793.25;
% a1 = .5258;
% a2 = .0480;
% a3 = .9560;
% a4 = 708.1229;
% a5 = 1.9591;
% a6 = 25.4768;
% a7 = -31.3957;
% a8 = 714.8015;
% a9 = 977.84;
% a1 = -.2489;
% a2 = -.0743;
% a3 = 2.0965;
% a4 = 10.7338;
% a5 = 9.7358;
% a6 = -.0814;
% a7 = 4.5641;
% a8 = 1.2481;
% a9 = -5.8646;
% a1 = -.2209;
% a2 = -.1179;
% a3 = 2.1619;
% a4 = 11.0577;
% a5 = 9.7756;
% a6 = .0600;
% a7 = -11.0331;
% a8 = 508.5979;
% a9 = 156.7023;
% a1 = .5634
% a2 = .0174
% a3 = .0665
% a4 = 5.6429
% a5 = 4.6985
% a6 = .0088
% a7 = .0793
% a8 = -5.4009
% a9 = 106.9327
%slip = slip/.4

Force1 = ((a2*Ffr1.^2+a3*Ffr1).*sin(a1*atan(((a4*sin(a5*atan(a6*Ffr1)))./((a2*Ffr1.^2+a3*Ffr1)*a1)).*((a1-(a7*Ffr1.^2+a8*Ffr1+a9)).*slip + ((a7*Ffr1.^2+a8*Ffr1+a9)./((a4*sin(a5*atan(a6*Ffr1)))./((a2*Ffr1.^2+a3*Ffr1)*a1))).*atan(((a4*sin(a5*atan(a6*Ffr1)))./((a2*Ffr1.^2+a3*Ffr1)*a1)).*slip)))));
Force2 = ((a2*Ffr2.^2+a3*Ffr2).*sin(a1*atan(((a4*sin(a5*atan(a6*Ffr2)))./((a2*Ffr2.^2+a3*Ffr2)*a1)).*((a1-(a7*Ffr2.^2+a8*Ffr2+a9)).*slip + ((a7*Ffr2.^2+a8*Ffr2+a9)./((a4*sin(a5*atan(a6*Ffr2)))./((a2*Ffr2.^2+a3*Ffr2)*a1))).*atan(((a4*sin(a5*atan(a6*Ffr2)))./((a2*Ffr2.^2+a3*Ffr2)*a1)).*slip)))));
Force3 = ((a2*Ffr3.^2+a3*Ffr3).*sin(a1*atan(((a4*sin(a5*atan(a6*Ffr3)))./((a2*Ffr3.^2+a3*Ffr3)*a1)).*((a1-(a7*Ffr3.^2+a8*Ffr3+a9)).*slip + ((a7*Ffr3.^2+a8*Ffr3+a9)./((a4*sin(a5*atan(a6*Ffr3)))./((a2*Ffr3.^2+a3*Ffr3)*a1))).*atan(((a4*sin(a5*atan(a6*Ffr3)))./((a2*Ffr3.^2+a3*Ffr3)*a1)).*slip)))));
Force4 = ((a2*Ffr4.^2+a3*Ffr4).*sin(a1*atan(((a4*sin(a5*atan(a6*Ffr4)))./((a2*Ffr4.^2+a3*Ffr4)*a1)).*((a1-(a7*Ffr4.^2+a8*Ffr4+a9)).*slip + ((a7*Ffr4.^2+a8*Ffr4+a9)./((a4*sin(a5*atan(a6*Ffr4)))./((a2*Ffr4.^2+a3*Ffr4)*a1))).*atan(((a4*sin(a5*atan(a6*Ffr4)))./((a2*Ffr4.^2+a3*Ffr4)*a1)).*slip)))));
Force5 = ((a2*Ffr5.^2+a3*Ffr5).*sin(a1*atan(((a4*sin(a5*atan(a6*Ffr5)))./((a2*Ffr5.^2+a3*Ffr5)*a1)).*((a1-(a7*Ffr5.^2+a8*Ffr5+a9)).*slip + ((a7*Ffr5.^2+a8*Ffr5+a9)./((a4*sin(a5*atan(a6*Ffr5)))./((a2*Ffr5.^2+a3*Ffr5)*a1))).*atan(((a4*sin(a5*atan(a6*Ffr5)))./((a2*Ffr5.^2+a3*Ffr5)*a1)).*slip)))));

== matlab function FrankSensingDiscreteEKF/State Estimation1/Subsystem1/MATLAB Function ==
  data: startflag input; Kkpre input; Pkpre input; VymeasIMU input; Kkpost output; pdot output; VymeasGPS input; rmeas input; res output; Vx input; SA input; x input; xdot output; Xcov input; Ycov input
function [Kkpost, pdot, res, xdot] = myEKF(startflag, Kkpre, Pkpre, VymeasIMU, VymeasGPS, rmeas, Vx, SA, x, Xcov, Ycov)

a = .3036;
b = .2484;
B = 10;
C = 1.6;
D = 73.1580;
E = 1;
Iz = 1;
Mv = 15.7;
delta = SA;




VyvarIMU = 200;
VyvarGPS = Xcov;
rvar = .00001;


Rk = [VyvarIMU 0          0;...     
      0        VyvarGPS   0;...
      0        0          rvar];  %Measurement noise covariance matrix
      

Qk = [.1     0;...
      0          .1]; % process noise covariance matrix

zk = [VymeasIMU; VymeasGPS; rmeas];


% Startup Initialization
if startflag == 0
    Kk = [0    0  0;...
          0    0  0];
    Pk = [.00001     0;...
          0          .000002]; % process noise covariance matrix

    x = [-0.014;-0.44];
      
else
    Kk = Kkpre
    Pk = Pkpre
end

hk = [x(1);x(1);x(2)];
Vy = x(1);
r = x(2);
% Prediction and measurement jacobian
Hk = [1 0;1 0;0 1];

Fkf = Fk(B,C,D,E,Iz,Mv,Vx,Vy,a,b,delta,r);
fkf = Xdot(B,C,D,E,Iz,Mv,Vx,Vy,a,b,delta,r);
res = zk-hk;
xdot = fkf+Kk*(res);
pdot = Fkf*Pk+Pk*Fkf'-Kk*Hk*Pk+Qk;
Kkpost = Pk*Hk'*inv(Rk);





% % Measurement Updates
% S = (Hk*Pk*Hk')+Rk;
% Kkpost = Pk*Hk'*inv(S)
% Pkpost = Pk-Kk*Hk*Pk
% res = zk-Hk
% xhat = Statest + Kkpost*(res)
% 
% % % State Estimate update
% pdot = Fkf'*Pkpost+Pkpost*Fkf'-Kkpost*Hk*Pkpost + Qk

== matlab function FrankSensingDiscreteEKF/State Estimation/Subsystem1/MATLAB Function1 ==
  data: t input; Slipflag output
function Slipflag = fcn(t)

if t == 0
    Slipflag = 0;
else
    Slipflag = 1;
end

t
